simulink model "loaded_motor_ss"  (R2021b)
settings: Solver=VariableStepAuto  StartTime=0.0  StopTime=2  RelTol=1e-3
undefined symbols (not defined in the file or in its folder): Km, Kp, P5_A2, P5_B2, P5_C2, P5_D2
libraries: cstblocks x4
settings Model: Creator=andre  LastModifiedBy=andre

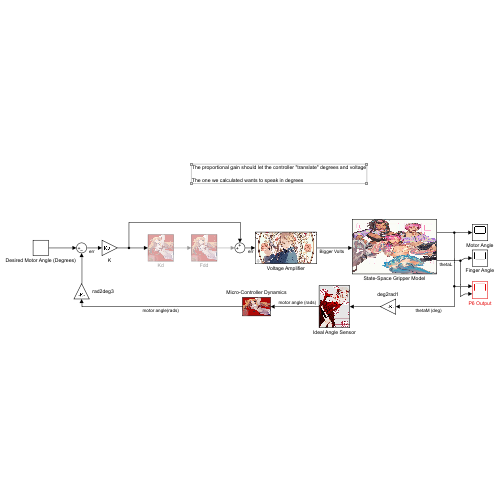
[thumbnail: Simulink's stored preview of the top-level diagram]
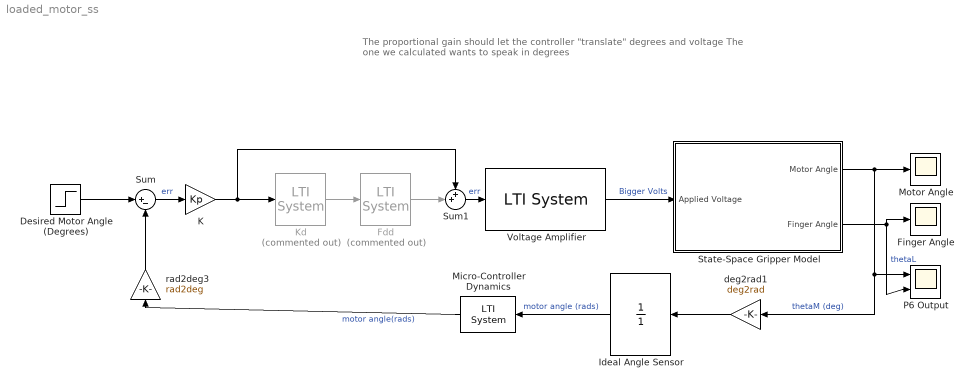
== system loaded_motor_ss ==
  note: The proportional gain should let the controller "translate" degrees and voltage
      |
      | The one we calculated wants to speak in degrees
  Desired Motor Angle (Degrees) : Step  Time=0  After=10  SampleTime=0
  Fdd : cstblocks/LTI System  Commented=on  sys=FDD  IC=[]  mask(LTI Block){}
      mask Display: image('X:\Pictures\Art\U91dtUSyLXXZLehty1jBZ2XQnwdifIIbPLO38neB02c.png'); % Use "Edit Image" on toolstrip to change.
  Finger Angle : Scope
  Ideal Angle Sensor : TransferFcn  Denominator=[1]
      mask Display: image('X:\Pictures\Art\EaVsDtGX0As3yGM.jpg'); % Use "Edit Image" on toolstrip to change.
  K : Gain  Gain=Kp
  Kd : cstblocks/LTI System  Commented=on  sys=KD  IC=[]  mask(LTI Block){}
      mask Display: image('X:\Pictures\Art\U91dtUSyLXXZLehty1jBZ2XQnwdifIIbPLO38neB02c.png'); % Use "Edit Image" on toolstrip to change.
  Micro-Controller Dynamics : cstblocks/LTI System  sys=mcu_dynamics  IC=[]  mask(LTI Block){}
      mask Display: image('X:\Pictures\Art\U91dtUSyLXXZLehty1jBZ2XQnwdifIIbPLO38neB02c.png'); % Use "Edit Image" on toolstrip to change.
  Motor Angle : Scope
  P6 Output : Scope  NumInputPorts=2
  State-Space Gripper Model : Subsystem
      mask Display: image('X:\Pictures\Art\EatYTXFU4AAE3UE.jpg'); % Use "Edit Image" on toolstrip to change.
  Sum : Sum  Inputs=|+-
  Sum1 : Sum  Inputs=++|
  Voltage Amplifier : cstblocks/LTI System  sys=P2_ampTF  IC=[]  mask(LTI Block){}
      mask Display: image('X:\Pictures\Art\EVz-gOfVAAARVVY.jpg'); % Use "Edit Image" on toolstrip to change.
  deg2rad1 : Gain  Gain=deg2rad
  rad2deg3 : Gain  Gain=rad2deg
  wires:
  Voltage Amplifier/1 -> State-Space Gripper Model/1(Applied Voltage)  "Bigger Volts"
  State-Space Gripper Model/1(" Motor Angle ") -> deg2rad1/1, P6 Output/1, Motor Angle/1  "thetaM (deg)"
  Micro-Controller Dynamics/1 -> rad2deg3/1  "motor angle(rads)"
  State-Space Gripper Model/2(" Finger Angle ") -> P6 Output/2, Finger Angle/1  "thetaL"
  Sum/1 -> K/1  "err"
  deg2rad1/1 -> Ideal Angle Sensor/1
  Ideal Angle Sensor/1 -> Micro-Controller Dynamics/1  "motor angle (rads)"
  Desired Motor Angle (Degrees)/1 -> Sum/1
  rad2deg3/1 -> Sum/2
  Kd/1 -> Fdd/1
  K/1 -> Kd/1, Sum1/1
  Fdd/1 -> Sum1/2
  Sum1/1 -> Voltage Amplifier/1  "err"

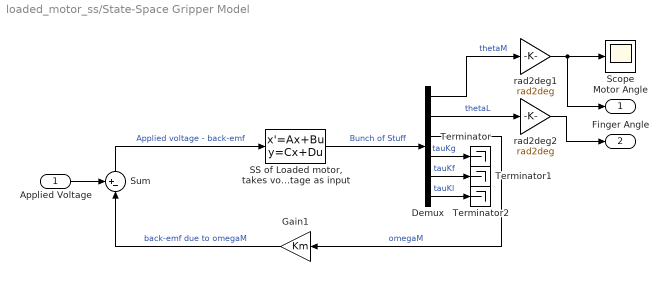
== system loaded_motor_ss/State-Space Gripper Model ==
  Applied Voltage : Inport
  Demux : Demux  Outputs=6
  Gain1 : Gain  Gain=Km
  "SS of Loaded motor, takes voltage as input" : StateSpace  A=P5_A2  B=P5_B2  C=P5_C2  D=P5_D2  InitialCondition=0  ParameterTunability=Unconstrained
  Scope : Scope
  Sum : Sum  Inputs=+-|
  Terminator : Terminator
  Terminator1 : Terminator
  Terminator2 : Terminator
  rad2deg1 : Gain  Gain=rad2deg
  rad2deg2 : Gain  Gain=rad2deg
  " Motor Angle " : Outport
  " Finger Angle " : Outport  Port=2
  wires:
  Demux/3 -> Gain1/1  "omegaM"
  Demux/5 -> Terminator1/1  "tauKf"
  Demux/6 -> Terminator2/1  "tauKl"
  rad2deg1/1 -> " Motor Angle "/1, Scope/1
  "SS of Loaded motor, takes voltage as input"/1 -> Demux/1  "Bunch of Stuff"
  Demux/4 -> Terminator/1  "tauKg"
  Gain1/1 -> Sum/2  "back-emf due to omegaM"
  Demux/1 -> rad2deg1/1  "thetaM"
  Demux/2 -> rad2deg2/1  "thetaL"
  Applied Voltage/1 -> Sum/1
  Sum/1 -> "SS of Loaded motor, takes voltage as input"/1  "Applied voltage - back-emf"
  rad2deg2/1 -> " Finger Angle "/1
